simulink model "global_sliding_mode"  (R2019b)
settings: Solver=VariableStepAuto  StartTime=0.0  StopTime=30  RelTol=1e-3
settings Model: Creator=Alien  LastModifiedBy=Alien

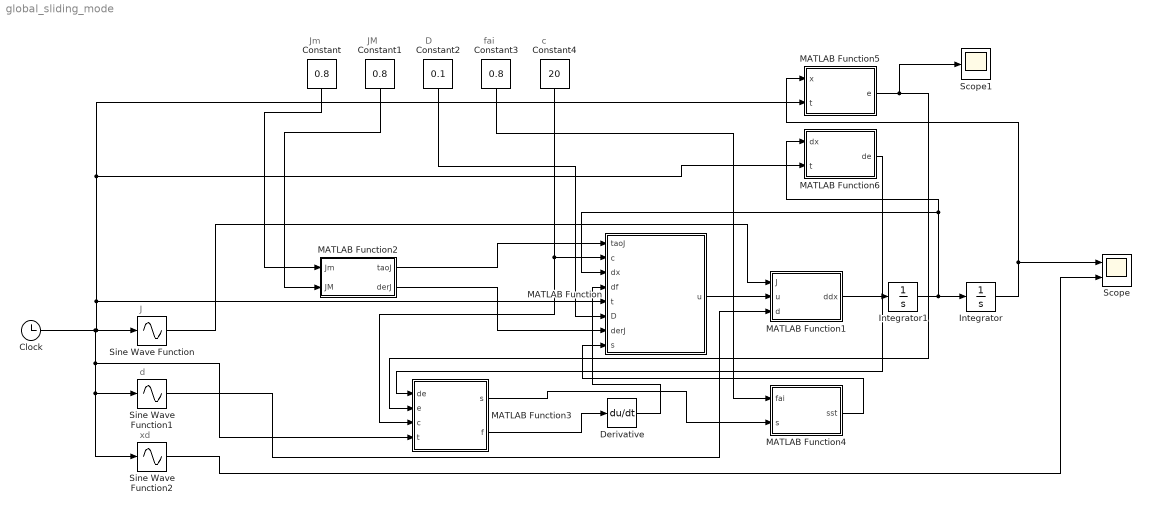
== system global_sliding_mode ==
  note: d
  note: J
  note: Jm
  note: JM
  note: D
  note: fai
  note: c
  note: xd
  Clock : Clock
  Constant : Constant  Value=0.8
  Constant1 : Constant  Value=0.8
  Constant2 : Constant  Value=0.1
  Constant3 : Constant  Value=0.8
  Constant4 : Constant  Value=20
  Derivative : Derivative
  Integrator : Integrator
  Integrator1 : Integrator
  MATLAB Function : MATLAB Function  TreatAsAtomicUnit=on
  MATLAB Function1 : MATLAB Function  TreatAsAtomicUnit=on
  MATLAB Function2 : MATLAB Function  TreatAsAtomicUnit=on
  MATLAB Function3 : MATLAB Function  TreatAsAtomicUnit=on
  MATLAB Function4 : MATLAB Function  TreatAsAtomicUnit=on
  MATLAB Function5 : MATLAB Function  TreatAsAtomicUnit=on
  MATLAB Function6 : MATLAB Function  TreatAsAtomicUnit=on
  Scope : Scope  NumInputPorts=2
  Scope1 : Scope
  Sine Wave Function : Sin  TimeSource=Use external signal  Amplitude=0.2  Bias=1  SampleTime=0
  Sine Wave Function1 : Sin  TimeSource=Use external signal  Amplitude=0.1  Frequency=2*pi  SampleTime=0
  Sine Wave Function2 : Sin  TimeSource=Use external signal  SampleTime=0
  wires:
  Integrator1/1 -> MATLAB Function6/1(dx), MATLAB Function/3(dx), Integrator/1
  MATLAB Function1/1(ddx) -> Integrator1/1
  MATLAB Function/1(u) -> MATLAB Function1/2(u)
  Constant/1 -> MATLAB Function2/1(Jm)
  Constant1/1 -> MATLAB Function2/2(JM)
  MATLAB Function2/1(taoJ) -> MATLAB Function/1(taoJ)
  MATLAB Function2/2(derJ) -> MATLAB Function/7(derJ)
  Constant4/1 -> MATLAB Function3/3(c), MATLAB Function/2(c)
  Derivative/1 -> MATLAB Function/4(df)
  Constant2/1 -> MATLAB Function/6(D)
  Integrator/1 -> MATLAB Function5/1(x), Scope/1
  MATLAB Function6/1(de) -> MATLAB Function3/1(de)
  MATLAB Function5/1(e) -> Scope1/1, MATLAB Function3/2(e)
  Clock/1 -> MATLAB Function3/4(t), Sine Wave Function2/1, Sine Wave Function1/1, MATLAB Function6/2(t), MATLAB Function5/2(t), MATLAB Function/5(t), Sine Wave Function/1
  Sine Wave Function/1 -> MATLAB Function1/1(J)
  Sine Wave Function1/1 -> MATLAB Function1/3(d)
  Sine Wave Function2/1 -> Scope/2
  MATLAB Function3/2(f) -> Derivative/1
  MATLAB Function3/1(s) -> MATLAB Function4/2(s)
  Constant3/1 -> MATLAB Function4/1(fai)
  MATLAB Function4/1(sst) -> MATLAB Function/8(s)

== matlab function global_sliding_mode/MATLAB Function1 ==
  data: J input; u input; ddx output; d input
function ddx = fcn(J, u, d)
ddx = 1/J*(u - d);

== matlab function global_sliding_mode/MATLAB Function ==
  data: taoJ input; u output; c input; dx input; df input; t input; D input; derJ input; s input
function u = fcn(taoJ, c, dx, df, t, D, derJ, s)
dxd = cos(t);
ddxd = -sin(t);
u = -taoJ*(c*dx - df) + taoJ*(ddxd + c*dxd) - (derJ*abs(c*dx - df) + D + derJ*(ddxd + c*dxd))*s;

== matlab function global_sliding_mode/MATLAB Function2 ==
  data: Jm input; taoJ output; JM input; derJ output
function [taoJ, derJ] = fcn(Jm, JM)
taoJ = (Jm + JM)/2;
derJ = (JM - Jm)/2;

== matlab function global_sliding_mode/MATLAB Function3 ==
  settings: updateMethod=DISCRETE
  data: de input; s output; e input; c input; t input; f output
function [s, f] = fcn(de, e, c, t)
persistent s0 ft;
if isempty(s0)
    s0 = 0;
    ft = 0;
end
s = de + c*e + ft;
if(t==0)
    s0 = s;
end
ft = s0*(exp(-130*t));
f = ft;

== matlab function global_sliding_mode/MATLAB Function4 ==
  data: fai input; sst output; s input
function sst = fcn(fai, s)
persistent jd;
jd = s/fai;
if(jd > 1)
    sst = 1;
elseif(jd < -1)
    sst = -1;
else
    sst = jd;
end

== matlab function global_sliding_mode/MATLAB Function5 ==
  data: x input; e output; t input
function e = fcn(x, t)
e = sin(t) - x;

== matlab function global_sliding_mode/MATLAB Function6 ==
  data: dx input; de output; t input
function de = fcn(dx, t)
de = cos(t) - dx;
